simulink library "deadRecPos_cl"  (R2020a)
settings: Solver=VariableStepAuto  StartTime=0.0  StopTime=10.0  RelTol=1e-3
values from neighbouring files (symbols this model uses):
  sns = SNS.realistic    [deadRecPos_bs.m]
undefined symbols (not defined in the file or in its folder): initializeBussesFromBlock
libraries: vrlib x4, dspsigops x4, simulink x2, eulAng2RotMat_ul x2
settings Model: Creator=mcobb  LastModifiedBy=adabney
settings DataIOCC: ReturnWorkspaceOutputs=off
settings DebuggingCC: ArithmeticOperatorsInVariantConditions=warning
settings SFSimCC: CustomCodeUndefinedFunction=UseInterfaceOnly

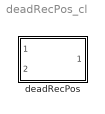
== system deadRecPos_cl ==
  deadRecPos : Subsystem  LoadFcn=initializeBussesFromBlock(gcb)  InitFcn=initializeBussesFromBlock(gcb)  StartFcn=initializeBussesFromBlock(gcb)

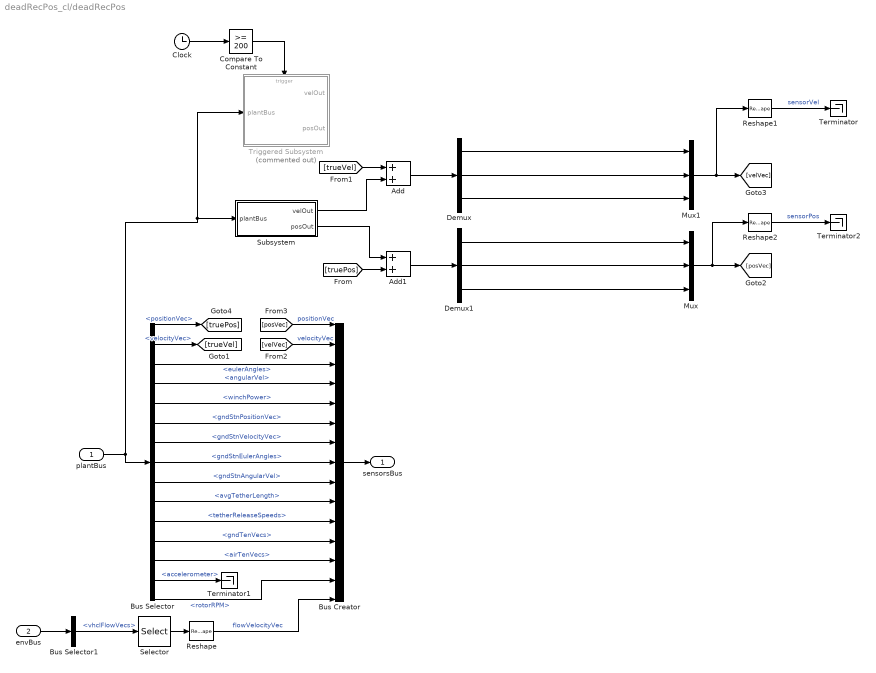
== system deadRecPos_cl/deadRecPos ==
  plantBus : Inport  OutDataTypeStr=Bus: plantBus
  envBus : Inport  Port=2  OutDataTypeStr=Bus: envBus
  Add : Sum
  Add1 : Sum
  Bus Creator : BusCreator  Inputs=15  OutDataTypeStr=Bus: sensorsBus  NonVirtualBus=on
  Bus Selector : BusSelector  OutputSignals=positionVec,velocityVec,eulerAngles,angularVel,winchPower,gndStnPositionVec,gndStnVelocityVec,gndStnEulerAngles,gndStnAngularVel,avgTetherLength,tetherReleaseSpeeds,gndTenVecs,airTenVecs,accelerometer,rotorRPM
  Bus Selector1 : BusSelector  OutputSignals=vhclFlowVecs
  Clock : Clock
  Compare To Constant : simulink/Logic and Bit Operations/Compare To Constant  relop=>=  const=200  OutDataTypeStr=boolean
  Demux : Demux  Outputs=3
  Demux1 : Demux  Outputs=3
  Mux : Mux  Inputs=3
  Mux1 : Mux  Inputs=3
  Reshape : Reshape  OutputDimensionality=Column vector (2-D)
  Reshape1 : Reshape  OutputDimensionality=Column vector (2-D)
  Reshape2 : Reshape  OutputDimensionality=Column vector (2-D)
  Selector : Selector  NumberOfDimensions=2  InputPortWidth=3  IndexOptions=Select all,Index vector (dialog)  Indices=[1 3],1  OutputSizes=1,1
  Subsystem : Subsystem
  Terminator : Terminator
  Terminator1 : Terminator
  Terminator2 : Terminator
  Triggered Subsystem : Subsystem  Commented=on  TreatAsAtomicUnit=on
  sensorsBus : Outport  OutDataTypeStr=Bus: sensorsBus  VectorParamsAs1DForOutWhenUnconnected=off
  wires:
  plantBus/1 -> Subsystem/1(plantBus), Triggered Subsystem/1(plantBus), Bus Selector/1
  envBus/1 -> Bus Selector1/1
  Bus Selector1/1 -> Selector/1  "<vhclFlowVecs>"
  Selector/1 -> Reshape/1
  Reshape/1 -> Bus Creator/15  "flowVelocityVec"
  Bus Creator/1 -> sensorsBus/1
  [posVec] -> Bus Creator/1  "positionVec"
  Bus Selector/12 -> Bus Creator/12  "<gndTenVecs>"
  [velVec] -> Bus Creator/2  "velocityVec"
  Bus Selector/3 -> Bus Creator/3  "<eulerAngles>"
  Bus Selector/4 -> Bus Creator/4  "<angularVel>"
  Bus Selector/5 -> Bus Creator/5  "<winchPower>"
  Bus Selector/6 -> Bus Creator/6  "<gndStnPositionVec>"
  Bus Selector/7 -> Bus Creator/7  "<gndStnVelocityVec>"
  Bus Selector/8 -> Bus Creator/8  "<gndStnEulerAngles>"
  Bus Selector/9 -> Bus Creator/9  "<gndStnAngularVel>"
  Bus Selector/10 -> Bus Creator/10  "<avgTetherLength>"
  Bus Selector/11 -> Bus Creator/11  "<tetherReleaseSpeeds>"
  Bus Selector/13 -> Bus Creator/13  "<airTenVecs>"
  Bus Selector/14 -> Terminator1/1  "<accelerometer>"
  Bus Selector/1 -> [truePos]  "<positionVec>"
  Bus Selector/2 -> [trueVel]  "<velocityVec>"
  Subsystem/2(posOut) -> Add1/1
  Subsystem/1(velOut) -> Add/2
  Bus Selector/15 -> Bus Creator/14  "<rotorRPM>"
  Clock/1 -> Compare To Constant/1
  Compare To Constant/1 -> Triggered Subsystem/Trigger
  Add/1 -> Demux/1
  [trueVel] -> Add/1
  [truePos] -> Add1/2
  Add1/1 -> Demux1/1
  Mux1/1 -> Reshape1/1, [velVec]
  Demux/1 -> Mux1/1
  Demux/2 -> Mux1/2
  Demux/3 -> Mux1/3
  Demux1/1 -> Mux/1
  Demux1/2 -> Mux/2
  Demux1/3 -> Mux/3
  Reshape1/1 -> Terminator/1  "sensorVel"
  Mux/1 -> Reshape2/1, [posVec]
  Reshape2/1 -> Terminator2/1  "sensorPos"

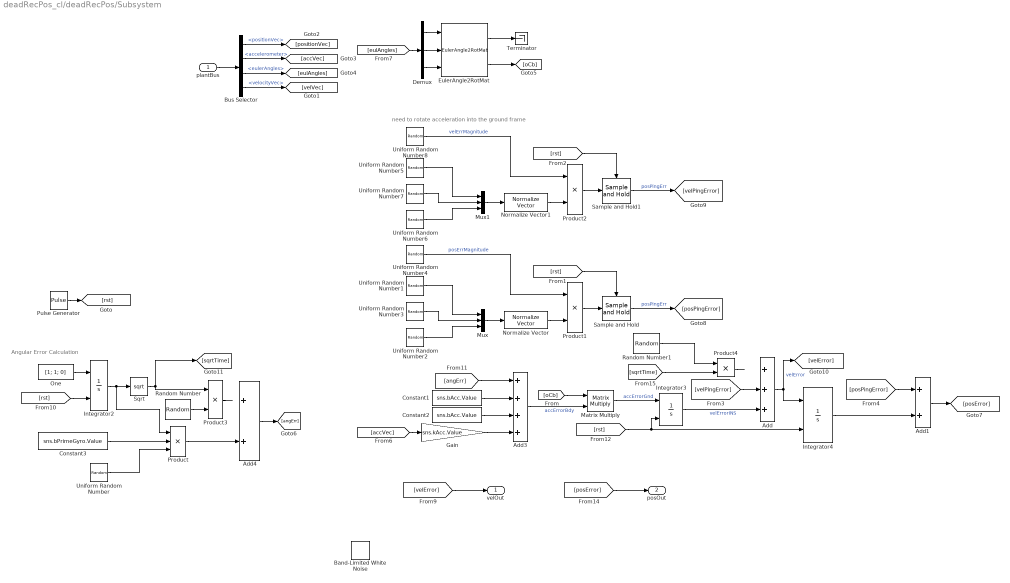
== system deadRecPos_cl/deadRecPos/Subsystem ==
  note: need to rotate acceleration into the ground frame
  note: Angular Error Calculation
  plantBus : Inport
  Add : Sum  Inputs=+++
  Add1 : Sum
  Add3 : Sum  Inputs=++++
  Add4 : Sum
  Band-Limited White Noise : simulink/Sources/Band-Limited White Noise  Cov=[0.1]  Ts=0.1  seed=[23341]
  Bus Selector : BusSelector  OutputSignals=positionVec,accelerometer,eulerAngles,velocityVec
  Constant1 : Constant  Value=sns.bAcc.Value
  Constant2 : Constant  Value=sns.bAcc.Value
  Constant3 : Constant  Value=sns.bPrimeGyro.Value
  Demux : Demux  Outputs=3
  EulerAngle2RotMat : eulAng2RotMat_ul/EulerAngle2RotMat  SystemSampleTime=-1  Latency=0  AutoFrameSizeCalculation=off
  Gain : Gain  Gain=sns.kAcc.Value
  Integrator2 : Integrator  ExternalReset=rising
  Integrator3 : Integrator  ExternalReset=rising
  Integrator4 : Integrator  ExternalReset=rising
  Matrix Multiply : Product  Multiplication=Matrix(*)
  Mux : Mux  Inputs=3
  Mux1 : Mux  Inputs=3
  Normalize Vector : vrlib/Utilities/Normalize Vector  maxzero=0
  Normalize Vector1 : vrlib/Utilities/Normalize Vector  maxzero=0
  One : Constant  Value=[1; 1; 0]  OutDataTypeStr=Inherit: Inherit via back propagation
  Product : Product  Inputs=3
  Product{1..4} (4 alike) : Product
  Pulse Generator : DiscretePulseGenerator  PulseType=Time based  Period=(sns.gndTruthFreq.Value/(2*pi))^-1  PulseWidth=5
  Random Number : RandomNumber  Variance=(sns.ARW.Value*sqrt(sns.gndTruthFreq.Value/(2*pi)))^2
  Random Number1 : RandomNumber  Variance=(sns.VRW.Value*sqrt(sns.gndTruthFreq.Value/(2*pi)))^2
  Sample and Hold : dspsigops/Sample and Hold  trig=Rising edge  initCond=0  latchinput=off
  Sample and Hold1 : dspsigops/Sample and Hold  trig=Rising edge  initCond=0  latchinput=off
  Sqrt : Sqrt  SaturateOnIntegerOverflow=on
  Terminator : Terminator
  Uniform Random Number : UniformRandomNumber  Minimum=0
  Uniform Random Number1 : UniformRandomNumber  Minimum=0
  Uniform Random Number2 : UniformRandomNumber  Minimum=0  Seed=78654
  Uniform Random Number3 : UniformRandomNumber  Minimum=0  Seed=2459
  Uniform Random Number4 : UniformRandomNumber  Minimum=0  Maximum=sns.posErrMag.Value
  Uniform Random Number5 : UniformRandomNumber  Minimum=0  Seed=1954
  Uniform Random Number6 : UniformRandomNumber  Minimum=0  Seed=3
  Uniform Random Number7 : UniformRandomNumber  Minimum=0  Seed=549
  Uniform Random Number8 : UniformRandomNumber  Minimum=0  Maximum=sns.velErrMag.Value
  velOut : Outport
  posOut : Outport  Port=2
  wires:
  [velPingError] -> Add/2
  [posError] -> posOut/1
  Random Number/1 -> Product3/2
  [rst] -> Integrator2/2
  [oCb] -> Matrix Multiply/1
  Integrator2/1 -> Product/1, Sqrt/1
  Integrator3/1 -> Add/3  "velErrorINS"
  [posPingError] -> Add1/1
  EulerAngle2RotMat/1 -> Terminator/1
  Product2/1 -> Sample and Hold1/1
  [rst] -> Integrator3/2, Integrator4/2
  [accVec] -> Gain/1
  Normalize Vector1/1 -> Product2/2
  Uniform Random Number7/1 -> Mux1/2
  Bus Selector/4 -> [velVec]  "<velocityVec>"
  Uniform Random Number6/1 -> Mux1/3
  [velError] -> velOut/1
  Mux1/1 -> Normalize Vector1/1
  [angErr] -> Add3/1
  Product1/1 -> Sample and Hold/1
  Product4/1 -> ?
  Integrator4/1 -> Add1/2
  Matrix Multiply/1 -> Integrator3/1  "accErrorGnd"
  Mux/1 -> Normalize Vector/1
  Uniform Random Number8/1 -> Product2/1  "velErrMagnitude"
  Uniform Random Number2/1 -> Mux/3
  [sqrtTime] -> Product4/2
  Normalize Vector/1 -> Product1/2
  Gain/1 -> Add3/4
  Constant1/1 -> Add3/2
  Random Number1/1 -> Product4/1
  [rst] -> Sample and Hold/Trigger
  Sample and Hold/1 -> [posPingError]  "posPingErr"
  Uniform Random Number3/1 -> Mux/2
  One/1 -> Integrator2/1
  Uniform Random Number/1 -> Product/3
  Pulse Generator/1 -> [rst]
  Constant2/1 -> Add3/3
  Add3/1 -> Matrix Multiply/2  "accErrorBdy"
  Add/1 -> [velError], Integrator4/1  "velError"
  Product3/1 -> ?
  Uniform Random Number4/1 -> Product1/1  "posErrMagnitude"
  Demux/3 -> EulerAngle2RotMat/3
  Uniform Random Number5/1 -> Mux1/1
  Bus Selector/2 -> [accVec]  "<accelerometer>"
  [eulAngles] -> Demux/1
  plantBus/1 -> Bus Selector/1
  Bus Selector/1 -> [positionVec]  "<positionVec>"
  Sample and Hold1/1 -> [velPingError]  "posPingErr"
  Sqrt/1 -> Product3/1, [sqrtTime]
  Add4/1 -> [angErr]
  Demux/1 -> EulerAngle2RotMat/1
  Constant3/1 -> Product/2
  Demux/2 -> EulerAngle2RotMat/2
  [rst] -> Sample and Hold1/Trigger
  EulerAngle2RotMat/2 -> [oCb]
  Bus Selector/3 -> [eulAngles]  "<eulerAngles>"
  Product/1 -> Add4/2
  Uniform Random Number1/1 -> Mux/1
  Add1/1 -> [posError]

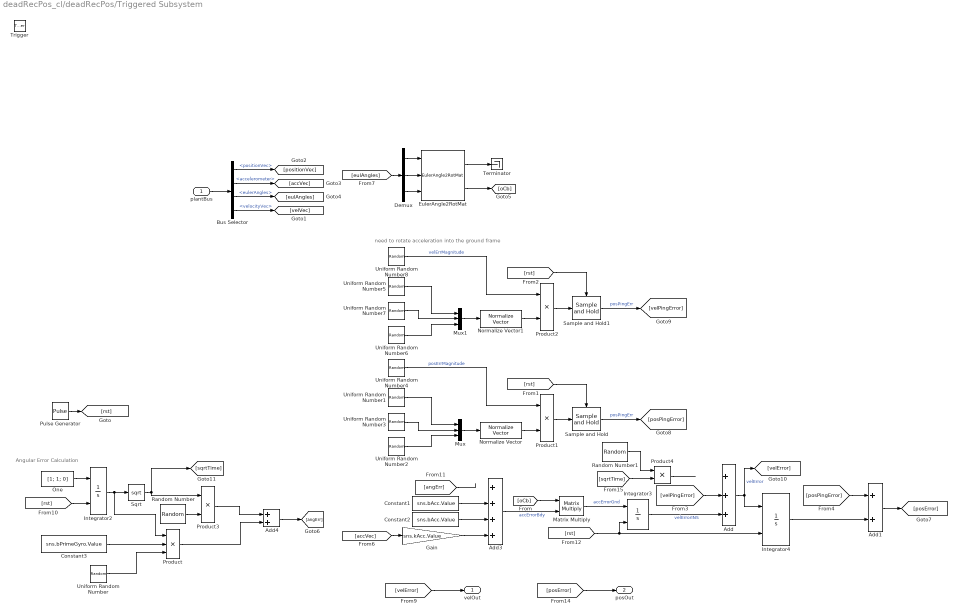
== system deadRecPos_cl/deadRecPos/Triggered Subsystem ==
  note: Angular Error Calculation
  note: need to rotate acceleration into the ground frame
  plantBus : Inport
  Trigger : TriggerPort  VariantControl=Variant
  Add : Sum  Inputs=+++
  Add1 : Sum
  Add3 : Sum  Inputs=++++
  Add4 : Sum
  Bus Selector : BusSelector  OutputSignals=positionVec,accelerometer,eulerAngles,velocityVec
  Constant1 : Constant  Value=sns.bAcc.Value
  Constant2 : Constant  Value=sns.bAcc.Value
  Constant3 : Constant  Value=sns.bPrimeGyro.Value
  Demux : Demux  Outputs=3
  EulerAngle2RotMat : eulAng2RotMat_ul/EulerAngle2RotMat  SystemSampleTime=-1  Latency=0  AutoFrameSizeCalculation=off
  Gain : Gain  Gain=sns.kAcc.Value
  Integrator2 : Integrator  ExternalReset=rising
  Integrator3 : Integrator  ExternalReset=rising
  Integrator4 : Integrator  ExternalReset=rising
  Matrix Multiply : Product  Multiplication=Matrix(*)
  Mux : Mux  Inputs=3
  Mux1 : Mux  Inputs=3
  Normalize Vector : vrlib/Utilities/Normalize Vector  maxzero=0
  Normalize Vector1 : vrlib/Utilities/Normalize Vector  maxzero=0
  One : Constant  Value=[1; 1; 0]  OutDataTypeStr=Inherit: Inherit via back propagation
  Product : Product  Inputs=3
  Product{1..4} (4 alike) : Product
  Pulse Generator : DiscretePulseGenerator  PulseType=Time based  Period=(sns.gndTruthFreq.Value/(2*pi))^-1  PulseWidth=5
  Random Number : RandomNumber  Variance=(sns.ARW.Value*sqrt(sns.gndTruthFreq.Value/(2*pi)))^2
  Random Number1 : RandomNumber  Variance=(sns.VRW.Value*sqrt(sns.gndTruthFreq.Value/(2*pi)))^2
  Sample and Hold : dspsigops/Sample and Hold  trig=Rising edge  initCond=0  latchinput=off
  Sample and Hold1 : dspsigops/Sample and Hold  trig=Rising edge  initCond=0  latchinput=off
  Sqrt : Sqrt  SaturateOnIntegerOverflow=on
  Terminator : Terminator
  Uniform Random Number : UniformRandomNumber  Minimum=0
  Uniform Random Number1 : UniformRandomNumber  Minimum=0
  Uniform Random Number2 : UniformRandomNumber  Minimum=0  Seed=78654
  Uniform Random Number3 : UniformRandomNumber  Minimum=0  Seed=2459
  Uniform Random Number4 : UniformRandomNumber  Minimum=0  Maximum=sns.posErrMag.Value
  Uniform Random Number5 : UniformRandomNumber  Minimum=0  Seed=1954
  Uniform Random Number6 : UniformRandomNumber  Minimum=0  Seed=3
  Uniform Random Number7 : UniformRandomNumber  Minimum=0  Seed=549
  Uniform Random Number8 : UniformRandomNumber  Minimum=0  Maximum=sns.velErrMag.Value
  velOut : Outport
  posOut : Outport  Port=2
  wires:
  [velError] -> velOut/1
  EulerAngle2RotMat/1 -> Terminator/1
  Random Number/1 -> Product3/2
  [posError] -> posOut/1
  [velPingError] -> Add/2
  Random Number1/1 -> Product4/1
  Uniform Random Number4/1 -> Product1/1  "posErrMagnitude"
  Constant1/1 -> Add3/2
  Gain/1 -> Add3/4
  [rst] -> Sample and Hold/Trigger
  Uniform Random Number2/1 -> Mux/3
  Normalize Vector/1 -> Product1/2
  Uniform Random Number8/1 -> Product2/1  "velErrMagnitude"
  Mux/1 -> Normalize Vector/1
  Matrix Multiply/1 -> Integrator3/1  "accErrorGnd"
  Integrator4/1 -> Add1/2
  Uniform Random Number1/1 -> Mux/1
  Product1/1 -> Sample and Hold/1
  Product4/1 -> ?
  [angErr] -> ?
  Mux1/1 -> Normalize Vector1/1
  [rst] -> Sample and Hold1/Trigger
  Constant2/1 -> Add3/3
  Normalize Vector1/1 -> Product2/2
  Uniform Random Number6/1 -> Mux1/3
  Add3/1 -> Matrix Multiply/2  "accErrorBdy"
  Uniform Random Number7/1 -> Mux1/2
  Sample and Hold1/1 -> [velPingError]  "posPingErr"
  Product2/1 -> Sample and Hold1/1
  [rst] -> Integrator3/2, Integrator4/2
  [posPingError] -> Add1/1
  [accVec] -> Gain/1
  Add4/1 -> [angErr]
  Bus Selector/4 -> [velVec]  "<velocityVec>"
  [oCb] -> Matrix Multiply/1
  Integrator3/1 -> Add/3  "velErrorINS"
  [rst] -> Integrator2/2
  Integrator2/1 -> Product/1, Sqrt/1
  One/1 -> Integrator2/1
  [sqrtTime] -> Product4/2
  Uniform Random Number3/1 -> Mux/2
  Sample and Hold/1 -> [posPingError]  "posPingErr"
  Product/1 -> Add4/2
  Constant3/1 -> Product/2
  Demux/2 -> EulerAngle2RotMat/2
  Sqrt/1 -> Product3/1, [sqrtTime]
  Demux/1 -> EulerAngle2RotMat/1
  Add1/1 -> [posError]
  EulerAngle2RotMat/2 -> [oCb]
  Bus Selector/3 -> [eulAngles]  "<eulerAngles>"
  Bus Selector/1 -> [positionVec]  "<positionVec>"
  Demux/3 -> EulerAngle2RotMat/3
  Bus Selector/2 -> [accVec]  "<accelerometer>"
  plantBus/1 -> Bus Selector/1
  Uniform Random Number/1 -> Product/3
  Pulse Generator/1 -> [rst]
  Add/1 -> [velError], Integrator4/1  "velError"
  [eulAngles] -> Demux/1
  Product3/1 -> Add4/1
  Uniform Random Number5/1 -> Mux1/1
